simulink model "WESDem_CalcState"  (R2016b)
settings: configuration reference "CodeGenConfigSet" (kept outside this file)
values from neighbouring files (symbols this model uses):
  WESDem_stCfg_C = Calibration.Parameter    [init_WESDem_CalcState.m]
  WESDem_stCfgvalid_C = Calibration.Parameter    [init_WESDem_CalcState.m]
  WESDem_stCrCtlInhibActv_C = Calibration.Parameter    [init_WESDem_CalcState.m]
  WESDem_stMode_C = Calibration.Parameter    [init_WESDem_CalcState.m]
  WESDem_stModevalid_C = Calibration.Parameter    [init_WESDem_CalcState.m]
  WESDem_swtEnaStrtModChng_C = Calibration.Parameter    [init_WESDem_CalcState.m]
  WESDem_tiBlockAftStrt_C = Calibration.Parameter    [init_WESDem_CalcState.m]
  WESDem_tiNeutr_C = Calibration.Parameter    [init_WESDem_CalcState.m]
  WESDem_trqThresNTC_C = Calibration.Parameter    [init_WESDem_CalcState.m]
  WESDem_vInhibCrCUI_C = Calibration.Parameter    [init_WESDem_CalcState.m]
  WESDem_vMaxAcc0_C = Calibration.Parameter    [init_WESDem_CalcState.m]
  WESDem_vMaxAcc1_C = Calibration.Parameter    [init_WESDem_CalcState.m]
  WESDem_vMaxAcc2_C = Calibration.Parameter    [init_WESDem_CalcState.m]
  WESDem_vMaxAcc3_C = Calibration.Parameter    [init_WESDem_CalcState.m]
undefined symbols (not defined in the file or in its folder): CrCUI_BttnState_conv, CruiseCtl_State_conv, EISGov_num_conv, EngState_conv, WESDem_CalcState_DT
libraries: simulink x50, CXLib x32
(part 1 of 2)
settings Model: Creator=zhoukai  LastModifiedBy=zhoukai
settings ConfigSetRef: SourceLocation=Base Workspace

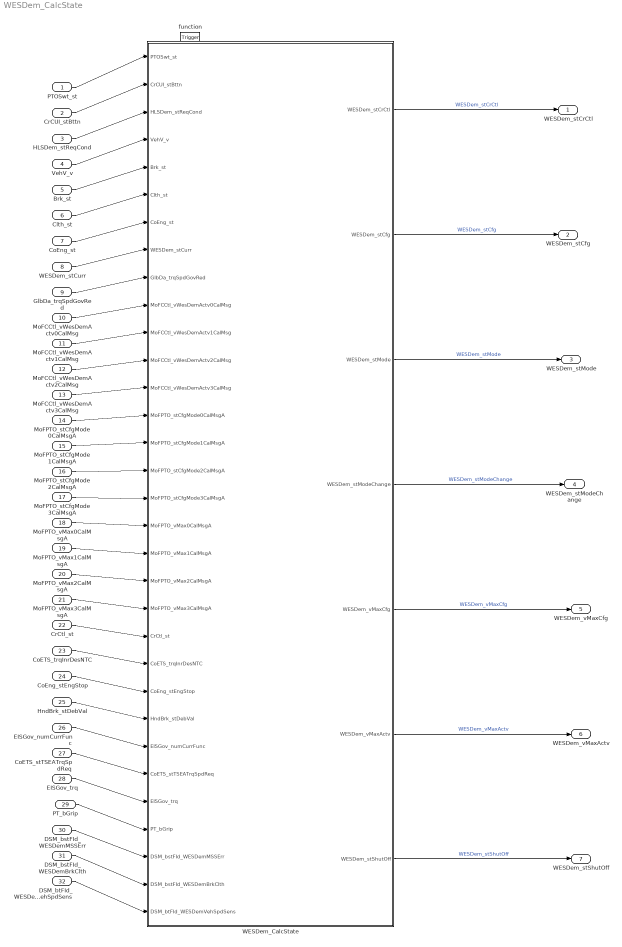
== system WESDem_CalcState ==
  PTOSwt_st : Inport  Description=Power Take-off switch's current state for a specific input voltage  OutMin=0  OutMax=255  OutDataTypeStr=State_uint8
  CrCUI_stBttn : Inport  Description=Application parameter for status button information  Port=2  OutDataTypeStr=Enum: CrCUI_BttnState_conv
  HLSDem_stReqCond : Inport  Description=Status of request for idle speed increase  Port=3  OutMin=0  OutMax=255  OutDataTypeStr=State_uint8
  VehV_v : Inport  Tag=km/h  Description=Vehicle speed  Port=4  OutMin=0  OutMax=250  OutDataTypeStr=VehSpeed_km_h
  Brk_st : Inport  Description=Brake switch state  Port=5  OutMin=0  OutMax=255  OutDataTypeStr=State_uint8
  Clth_st : Inport  Description=Clutch information  Port=6  OutMin=0  OutMax=255  OutDataTypeStr=State_uint8
  CoEng_st : Inport  Description=Engine coordinator state  Port=7  OutDataTypeStr=Enum: EngState_conv
  WESDem_stCurr : Inport  Description=Status of the working engine Speed Control  Port=8  OutDataTypeStr=Enum: WESDem_State_conv
  GlbDa_trqSpdGovRed : Inport  Tag=Nm  Description=Application parameter for negative torque threshold for the engine speed governor to be considered active.  Port=9  OutMin=-3276.8  OutMax=3276.7  OutDataTypeStr=Trq_Nm
  MoFCCtl_vWesDemActv0CalMsg : Inport  Tag=km/h  Description=MoFCCtl_vWesDemActvCalMsg[0]  Port=10  OutMin=0  OutMax=255  OutDataTypeStr=VehSpeed_km_h
  MoFCCtl_vWesDemActv1CalMsg : Inport  Tag=km/h  Description=MoFCCtl_vWesDemActvCalMsg[1]  Port=11  OutMin=0  OutMax=255  OutDataTypeStr=VehSpeed_km_h
  MoFCCtl_vWesDemActv2CalMsg : Inport  Tag=km/h  Description=MoFCCtl_vWesDemActvCalMsg[2]  Port=12  OutMin=0  OutMax=255  OutDataTypeStr=VehSpeed_km_h
  MoFCCtl_vWesDemActv3CalMsg : Inport  Tag=km/h  Description=MoFCCtl_vWesDemActvCalMsg[3]  Port=13  OutMin=0  OutMax=255  OutDataTypeStr=VehSpeed_km_h
  MoFPTO_stCfgMode0CalMsgA : Inport  Description=MoFPTO_stCfgModeCalMsgA[0]  Port=14  OutMin=0  OutMax=65535  OutDataTypeStr=State_uint16
  MoFPTO_stCfgMode1CalMsgA : Inport  Description=MoFPTO_stCfgModeCalMsgA[1]  Port=15  OutMin=0  OutMax=65535  OutDataTypeStr=State_uint16
  MoFPTO_stCfgMode2CalMsgA : Inport  Description=MoFPTO_stCfgModeCalMsgA[2]  Port=16  OutMin=0  OutMax=65535  OutDataTypeStr=State_uint16
  MoFPTO_stCfgMode3CalMsgA : Inport  Description=MoFPTO_stCfgModeCalMsgA[3]  Port=17  OutMin=0  OutMax=65535  OutDataTypeStr=State_uint16
  MoFPTO_vMax0CalMsgA : Inport  Tag=km/h  Description=MoFPTO_vMaxCalMsgA[0]  Port=18  OutMin=0  OutMax=250  OutDataTypeStr=VehSpeed_km_h
  MoFPTO_vMax1CalMsgA : Inport  Tag=km/h  Description=MoFPTO_vMaxCalMsgA[1]  Port=19  OutMin=0  OutMax=250  OutDataTypeStr=VehSpeed_km_h
  MoFPTO_vMax2CalMsgA : Inport  Tag=km/h  Description=MoFPTO_vMaxCalMsgA[2]  Port=20  OutMin=0  OutMax=250  OutDataTypeStr=VehSpeed_km_h
  MoFPTO_vMax3CalMsgA : Inport  Tag=km/h  Description=MoFPTO_vMaxCalMsgA[3]  Port=21  OutMin=0  OutMax=250  OutDataTypeStr=VehSpeed_km_h
  CrCtl_st : Inport  Description=Application parameter for Cruise Control state  Port=22  OutDataTypeStr=Enum: CruiseCtl_State_conv
  CoETS_trqInrDesNTC : Inport  Tag=Nm  Description=Additional desired engine friction Nm  Port=23  OutMin=-3276  OutMax=3276  OutDataTypeStr=Trq_Nm
  CoEng_stEngStop : Inport  Description=Bit coded output message from engine stop function for low idle, egine shut off and crank control  Port=24  OutMin=0  OutMax=255  OutDataTypeStr=State_uint8
  HndBrk_stDebVal : Inport  Description=Debounced value of Hand Brake switch  Port=25  OutMin=0  OutMax=255  OutDataTypeStr=State_uint8
  EISGov_numCurrFunc : Inport  Description=Identification name / number of the currently active EISGov client, which determines the current controller parameters  Port=26  OutDataTypeStr=Enum: EISGov_num_conv
  CoETS_stTSEATrqSpdReq : Inport  Description=Status of information about torque and speed intervention  Port=27  OutMin=0  OutMax=65535  OutDataTypeStr=State_uint16
  EISGov_trq : Inport  Tag=Nm  Description=Resulted output torque of EISGov controller  Port=28  OutMin=-3276.8  OutMax=3276.7  OutDataTypeStr=Trq_Nm
  PT_bGrip : Inport  Description=Grip is for sure present (the converter lockup clutch / the automated or manual clutch is completely closed and PT_bNoGrip = FALSE)  Port=29  OutMin=0  OutMax=1  OutDataTypeStr=boolean
  DSM_bstFId_WESDemMSSErr : Inport  Description=Function Identifier for WESDem reactions in case of multiple state switch error  Port=30  OutMin=0  OutMax=1  OutDataTypeStr=boolean
  DSM_bstFId_WESDemBrkClth : Inport  Description=FId inhibits if brake or clutch is faulty  Port=31  OutMin=0  OutMax=1  OutDataTypeStr=boolean
  DSM_btFId_WESDemVehSpdSens : Inport  Description=Function Identifier for WESDem reactions in case of vehicle speed sensing error  Port=32  OutMin=0  OutMax=1  OutDataTypeStr=boolean
  function : TriggerPort  TriggerType=function-call  VariantControl=Variant
  WESDem_CalcState : Subsystem
  WESDem_stCrCtl : Outport  Description=State control of the working engine speed demand  OutMin=0  OutMax=65535  OutDataTypeStr=State_uint16
  WESDem_stCfg : Outport  Description=Configuration of the actual operating mode  Port=2  OutMin=0  OutMax=65535  OutDataTypeStr=State_uint16
  WESDem_stMode : Outport  Description=Operating mode of the working engine speed demand  Port=3  OutMin=0  OutMax=255  OutDataTypeStr=State_uint8
  WESDem_stModeChange : Outport  Description=Operating mode change of the working engine speed demand  Port=4  OutMin=0  OutMax=255  OutDataTypeStr=State_uint8
  WESDem_vMaxCfg : Outport  Tag=km/h  Description=Maximum speed for activation in the actual operating mode  Port=5  OutMin=0  OutMax=255  OutDataTypeStr=VehSpeed_km_h
  WESDem_vMaxActv : Outport  Tag=km/h  Description=Vehicle speed threshold for activation of the WESDem  Port=6  OutMin=0  OutMax=255  OutDataTypeStr=VehSpeed_km_h
  WESDem_stShutOff : Outport  Description=Shut off conditions for the Working engine speed Demand  Port=7  OutMin=0  OutMax=65535  OutDataTypeStr=State_uint16
  wires:
  PTOSwt_st/1 -> WESDem_CalcState/1(PTOSwt_st)
  CrCUI_stBttn/1 -> WESDem_CalcState/2(CrCUI_stBttn)
  HLSDem_stReqCond/1 -> WESDem_CalcState/3(HLSDem_stReqCond)
  VehV_v/1 -> WESDem_CalcState/4(VehV_v)
  Brk_st/1 -> WESDem_CalcState/5(Brk_st)
  Clth_st/1 -> WESDem_CalcState/6(Clth_st)
  CoEng_st/1 -> WESDem_CalcState/7(CoEng_st)
  WESDem_stCurr/1 -> WESDem_CalcState/8(WESDem_stCurr)
  GlbDa_trqSpdGovRed/1 -> WESDem_CalcState/9(GlbDa_trqSpdGovRed)
  MoFCCtl_vWesDemActv0CalMsg/1 -> WESDem_CalcState/10(MoFCCtl_vWesDemActv0CalMsg)
  MoFCCtl_vWesDemActv1CalMsg/1 -> WESDem_CalcState/11(MoFCCtl_vWesDemActv1CalMsg)
  MoFCCtl_vWesDemActv2CalMsg/1 -> WESDem_CalcState/12(MoFCCtl_vWesDemActv2CalMsg)
  MoFCCtl_vWesDemActv3CalMsg/1 -> WESDem_CalcState/13(MoFCCtl_vWesDemActv3CalMsg)
  MoFPTO_stCfgMode0CalMsgA/1 -> WESDem_CalcState/14(MoFPTO_stCfgMode0CalMsgA)
  MoFPTO_stCfgMode1CalMsgA/1 -> WESDem_CalcState/15(MoFPTO_stCfgMode1CalMsgA)
  MoFPTO_stCfgMode2CalMsgA/1 -> WESDem_CalcState/16(MoFPTO_stCfgMode2CalMsgA)
  MoFPTO_stCfgMode3CalMsgA/1 -> WESDem_CalcState/17(MoFPTO_stCfgMode3CalMsgA)
  MoFPTO_vMax0CalMsgA/1 -> WESDem_CalcState/18(MoFPTO_vMax0CalMsgA)
  MoFPTO_vMax1CalMsgA/1 -> WESDem_CalcState/19(MoFPTO_vMax1CalMsgA)
  MoFPTO_vMax2CalMsgA/1 -> WESDem_CalcState/20(MoFPTO_vMax2CalMsgA)
  MoFPTO_vMax3CalMsgA/1 -> WESDem_CalcState/21(MoFPTO_vMax3CalMsgA)
  CrCtl_st/1 -> WESDem_CalcState/22(CrCtl_st)
  CoETS_trqInrDesNTC/1 -> WESDem_CalcState/23(CoETS_trqInrDesNTC)
  CoEng_stEngStop/1 -> WESDem_CalcState/24(CoEng_stEngStop)
  HndBrk_stDebVal/1 -> WESDem_CalcState/25(HndBrk_stDebVal)
  EISGov_numCurrFunc/1 -> WESDem_CalcState/26(EISGov_numCurrFunc)
  CoETS_stTSEATrqSpdReq/1 -> WESDem_CalcState/27(CoETS_stTSEATrqSpdReq)
  EISGov_trq/1 -> WESDem_CalcState/28(EISGov_trq)
  PT_bGrip/1 -> WESDem_CalcState/29(PT_bGrip)
  WESDem_CalcState/1(WESDem_stCrCtl) -> WESDem_stCrCtl/1  "WESDem_stCrCtl"
  WESDem_CalcState/2(WESDem_stCfg) -> WESDem_stCfg/1  "WESDem_stCfg"
  WESDem_CalcState/3(WESDem_stMode) -> WESDem_stMode/1  "WESDem_stMode"
  WESDem_CalcState/4(WESDem_stModeChange) -> WESDem_stModeChange/1  "WESDem_stModeChange"
  WESDem_CalcState/5(WESDem_vMaxCfg) -> WESDem_vMaxCfg/1  "WESDem_vMaxCfg"
  WESDem_CalcState/6(WESDem_vMaxActv) -> WESDem_vMaxActv/1  "WESDem_vMaxActv"
  WESDem_CalcState/7(WESDem_stShutOff) -> WESDem_stShutOff/1  "WESDem_stShutOff"
  DSM_bstFId_WESDemMSSErr/1 -> WESDem_CalcState/30("DSM_bstFId_WESDemMSSErr ")
  DSM_bstFId_WESDemBrkClth/1 -> WESDem_CalcState/31("DSM_bstFId_WESDemBrkClth ")
  DSM_btFId_WESDemVehSpdSens/1 -> WESDem_CalcState/32("DSM_btFId_WESDemVehSpdSens ")

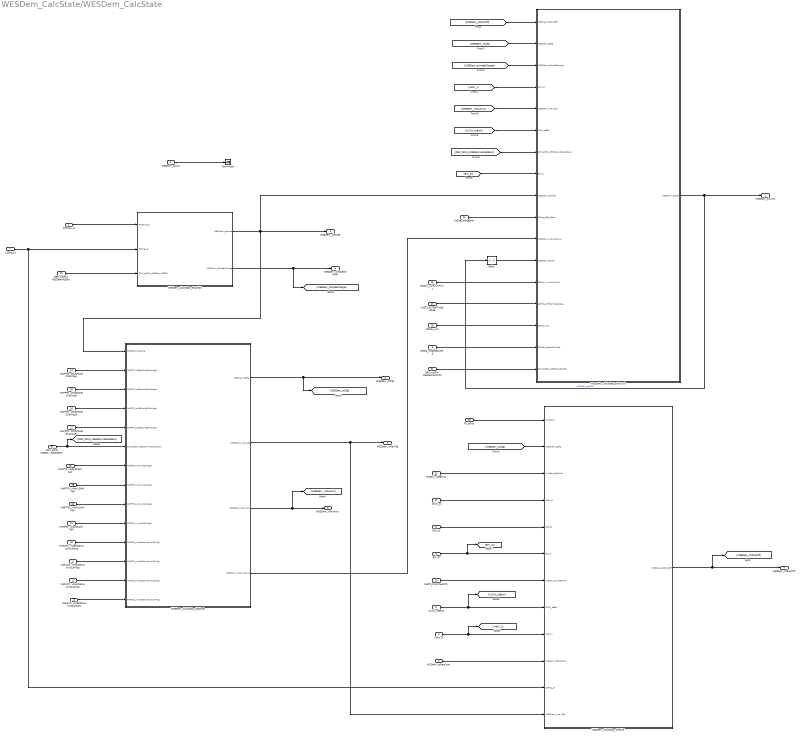
== system WESDem_CalcState/WESDem_CalcState ==
  PTOSwt_st : Inport  Description=Power Take-off switch's current state for a specific input voltage  OutMin=0  OutMax=255  OutDataTypeStr=State_uint8
  CrCUI_stBttn : Inport  Description=Application parameter for status button information  Port=2
  HLSDem_stReqCond : Inport  Description=Status of request for idle speed increase  Port=3  OutMin=0  OutMax=255  OutDataTypeStr=State_uint8
  VehV_v : Inport  Tag=km/h  Description=Vehicle speed  Port=4  OutMin=0  OutMax=250  OutDataTypeStr=VehSpeed_km_h
  Brk_st : Inport  Description=Brake switch state  Port=5  OutMin=0  OutMax=255  OutDataTypeStr=State_uint8
  Clth_st : Inport  Description=Clutch information  Port=6  OutMin=0  OutMax=255  OutDataTypeStr=State_uint8
  CoEng_st : Inport  Description=Engine coordinator state  Port=7  OutDataTypeStr=Enum: EngState_conv
  WESDem_stCurr : Inport  Description=Status of the working engine Speed Control  Port=8  OutDataTypeStr=Enum: WESDem_State_conv
  GlbDa_trqSpdGovRed : Inport  Tag=Nm  Description=Application parameter for negative torque threshold for the engine speed governor to be considered active.  Port=9  OutMin=-3276.8  OutMax=3276.7  OutDataTypeStr=Trq_Nm
  MoFCCtl_vWesDemActv0CalMsg : Inport  Tag=km/h  Description=MoFCCtl_vWesDemActvCalMsg[0]  Port=10  OutMin=0  OutMax=255  OutDataTypeStr=VehSpeed_km_h
  MoFCCtl_vWesDemActv1CalMsg : Inport  Tag=km/h  Description=MoFCCtl_vWesDemActvCalMsg[1]  Port=11  OutMin=0  OutMax=255  OutDataTypeStr=VehSpeed_km_h
  MoFCCtl_vWesDemActv2CalMsg : Inport  Tag=km/h  Description=MoFCCtl_vWesDemActvCalMsg[2]  Port=12  OutMin=0  OutMax=255  OutDataTypeStr=VehSpeed_km_h
  MoFCCtl_vWesDemActv3CalMsg : Inport  Tag=km/h  Description=MoFCCtl_vWesDemActvCalMsg[3]  Port=13  OutMin=0  OutMax=255  OutDataTypeStr=VehSpeed_km_h
  MoFPTO_stCfgMode0CalMsgA : Inport  Description=MoFPTO_stCfgModeCalMsgA[0]  Port=14  OutMin=0  OutMax=65535  OutDataTypeStr=State_uint16
  MoFPTO_stCfgMode1CalMsgA : Inport  Description=MoFPTO_stCfgModeCalMsgA[1]  Port=15  OutMin=0  OutMax=65535  OutDataTypeStr=State_uint16
  MoFPTO_stCfgMode2CalMsgA : Inport  Description=MoFPTO_stCfgModeCalMsgA[2]  Port=16  OutMin=0  OutMax=65535  OutDataTypeStr=State_uint16
  MoFPTO_stCfgMode3CalMsgA : Inport  Description=MoFPTO_stCfgModeCalMsgA[3]  Port=17  OutMin=0  OutMax=65535  OutDataTypeStr=State_uint16
  MoFPTO_vMax0CalMsgA : Inport  Tag=km/h  Description=MoFPTO_vMaxCalMsgA[0]  Port=18  OutMin=0  OutMax=250  OutDataTypeStr=VehSpeed_km_h
  MoFPTO_vMax1CalMsgA : Inport  Tag=km/h  Description=MoFPTO_vMaxCalMsgA[1]  Port=19  OutMin=0  OutMax=250  OutDataTypeStr=VehSpeed_km_h
  MoFPTO_vMax2CalMsgA : Inport  Tag=km/h  Description=MoFPTO_vMaxCalMsgA[2]  Port=20  OutMin=0  OutMax=250  OutDataTypeStr=VehSpeed_km_h
  MoFPTO_vMax3CalMsgA : Inport  Tag=km/h  Description=MoFPTO_vMaxCalMsgA[3]  Port=21  OutMin=0  OutMax=250  OutDataTypeStr=VehSpeed_km_h
  CrCtl_st : Inport  Description=Application parameter for Cruise Control state  Port=22
  CoETS_trqInrDesNTC : Inport  Tag=Nm  Description=Additional desired engine friction Nm  Port=23  OutMin=-3276  OutMax=3276  OutDataTypeStr=Trq_Nm
  CoEng_stEngStop : Inport  Description=Bit coded output message from engine stop function for low idle, egine shut off and crank control  Port=24  OutMin=0  OutMax=255  OutDataTypeStr=State_uint8
  HndBrk_stDebVal : Inport  Description=Debounced value of Hand Brake switch  Port=25  OutMin=0  OutMax=255  OutDataTypeStr=State_uint8
  EISGov_numCurrFunc : Inport  Description=Identification name / number of the currently active EISGov client, which determines the current controller parameters  Port=26  OutDataTypeStr=Enum: EISGov_num_conv
  CoETS_stTSEATrqSpdReq : Inport  Description=Status of information about torque and speed intervention  Port=27  OutMin=0  OutMax=65535  OutDataTypeStr=State_uint16
  EISGov_trq : Inport  Tag=Nm  Description=Resulted output torque of EISGov controller  Port=28  OutMin=-3276.8  OutMax=3276.7  OutDataTypeStr=Trq_Nm
  PT_bGrip : Inport  Description=Grip is for sure present (the converter lockup clutch / the automated or manual clutch is completely closed and PT_bNoGrip = FALSE)  Port=29  OutMin=0  OutMax=1  OutDataTypeStr=boolean
  "DSM_bstFId_WESDemMSSErr " : Inport  Description=Function Identifier for WESDem reactions in case of multiple state switch error  Port=30  OutMin=0  OutMax=1  OutDataTypeStr=boolean
  "DSM_bstFId_WESDemBrkClth " : Inport  Description=FId inhibits if brake or clutch is faulty  Port=31  OutMin=0  OutMax=1  OutDataTypeStr=boolean
  "DSM_btFId_WESDemVehSpdSens " : Inport  Description=Function Identifier for WESDem reactions in case of vehicle speed sensing error  Port=32  OutMin=0  OutMax=1  OutDataTypeStr=boolean
  Delay : Delay  DelayLength=1  InitialCondition=0
  Terminator : Terminator
  WESDem_CalcState_CfgMode : Subsystem
  WESDem_CalcState_EvalCrCtl : Subsystem
  WESDem_CalcState_EvalMSS : Subsystem
  WESDem_CalcState_ShutOff : Subsystem
  WESDem_stCrCtl : Outport  Description=State control of the working engine speed demand  OutMin=0  OutMax=65535  OutDataTypeStr=State_uint16
  WESDem_stCfg : Outport  Description=Configuration of the actual operating mode  Port=2  OutMin=0  OutMax=65535  OutDataTypeStr=State_uint16
  WESDem_stMode : Outport  Description=Operating mode of the working engine speed demand  Port=3  OutMin=0  OutMax=255  OutDataTypeStr=State_uint8
  WESDem_stModeChange : Outport  Description=Operating mode change of the working engine speed demand  Port=4  OutMin=0  OutMax=255  OutDataTypeStr=State_uint8
  WESDem_vMaxCfg : Outport  Description=Maximum speed for activation in the actual operating mode  Port=5  OutMin=0  OutMax=255  OutDataTypeStr=VehSpeed_km_h
  WESDem_vMaxActv : Outport  Description=Vehicle speed threshold for activation of the WESDem  Port=6  OutMin=0  OutMax=255  OutDataTypeStr=VehSpeed_km_h
  WESDem_stShutOff : Outport  Description=Shut off conditions for the Working engine speed Demand  Port=7  OutMin=0  OutMax=65535  OutDataTypeStr=State_uint16
  wires:
  WESDem_CalcState_EvalCrCtl/1(WESDem_stCrCtl) -> Delay/1, WESDem_stCrCtl/1  "WESDem_stCrCtl"
  PTOSwt_st/1 -> WESDem_CalcState_EvalMSS/1(PTOSwt_st)
  WESDem_CalcState_EvalMSS/2(WESDem_stModeChange) -> [WESDem_stModeChange], WESDem_stModeChange/1
  MoFPTO_stCfgMode0CalMsgA/1 -> WESDem_CalcState_CfgMode/2(MoFPTO_stCfgMode0CalMsgA)
  MoFPTO_stCfgMode1CalMsgA/1 -> WESDem_CalcState_CfgMode/3(MoFPTO_stCfgMode1CalMsgA)
  MoFPTO_stCfgMode2CalMsgA/1 -> WESDem_CalcState_CfgMode/4(MoFPTO_stCfgMode2CalMsgA)
  MoFPTO_stCfgMode3CalMsgA/1 -> WESDem_CalcState_CfgMode/5(MoFPTO_stCfgMode3CalMsgA)
  "DSM_btFId_WESDemVehSpdSens "/1 -> [DSM_btFId_WESDemVehSpdSens], WESDem_CalcState_CfgMode/6("DSM_btFId_WESDemVehSpdSens ")
  MoFPTO_vMax0CalMsgA/1 -> WESDem_CalcState_CfgMode/7(MoFPTO_vMax0CalMsgA)
  MoFPTO_vMax1CalMsgA/1 -> WESDem_CalcState_CfgMode/8(MoFPTO_vMax1CalMsgA)
  MoFPTO_vMax2CalMsgA/1 -> WESDem_CalcState_CfgMode/9(MoFPTO_vMax2CalMsgA)
  MoFPTO_vMax3CalMsgA/1 -> WESDem_CalcState_CfgMode/10(MoFPTO_vMax3CalMsgA)
  MoFCCtl_vWesDemActv0CalMsg/1 -> WESDem_CalcState_CfgMode/11(MoFCCtl_vWesDemActv0CalMsg)
  MoFCCtl_vWesDemActv1CalMsg/1 -> WESDem_CalcState_CfgMode/12(MoFCCtl_vWesDemActv1CalMsg)
  MoFCCtl_vWesDemActv2CalMsg/1 -> WESDem_CalcState_CfgMode/13(MoFCCtl_vWesDemActv2CalMsg)
  MoFCCtl_vWesDemActv3CalMsg/1 -> WESDem_CalcState_CfgMode/14(MoFCCtl_vWesDemActv3CalMsg)
  WESDem_CalcState_CfgMode/1(WESDem_stCfg) -> [WESDem_stCfg], WESDem_stCfg/1
  WESDem_CalcState_CfgMode/2(WESDem_vMaxCfg) -> WESDem_CalcState_ShutOff/12(WESDem_vMaxCfg), WESDem_vMaxCfg/1
  WESDem_CalcState_CfgMode/3(WESDem_vMaxActv) -> [WESDem_vMaxActv], WESDem_vMaxActv/1
  WESDem_CalcState_EvalMSS/1(WESDem_stMode) -> WESDem_CalcState_EvalCrCtl/9("WESDem_stMode "), WESDem_CalcState_CfgMode/1(WESDem_stMode), WESDem_stMode/1
  CoEng_st/1 -> WESDem_CalcState_ShutOff/11(CoEng_st), WESDem_CalcState_EvalMSS/2(CoEng_st)
  HndBrk_stDebVal/1 -> WESDem_CalcState_ShutOff/3(HndBrk_stDebVal)
  CrCtl_st/1 -> WESDem_CalcState_ShutOff/4(CrCtl_st)
  Clth_st/1 -> WESDem_CalcState_ShutOff/5(Clth_st)
  Brk_st/1 -> [Brk_st], WESDem_CalcState_ShutOff/6(Brk_st)
  CoETS_trqInrDesNTC/1 -> WESDem_CalcState_ShutOff/7(CoETS_trqInrDesNTC)
  CrCUI_stBttn/1 -> [CrCUI_stBttn], WESDem_CalcState_ShutOff/8(CrCUI_stBttn)
  VehV_v/1 -> [VehV_v], WESDem_CalcState_ShutOff/9(VehV_v)
  HLSDem_stReqCond/1 -> WESDem_CalcState_ShutOff/10(HLSDem_stReqCond)
  WESDem_CalcState_ShutOff/1(WESDem_stShutOff) -> [WESDem_stShutOff], WESDem_stShutOff/1
  PT_bGrip/1 -> WESDem_CalcState_ShutOff/1(PT_bGrip)
  GlbDa_trqSpdGovRed/1 -> WESDem_CalcState_EvalCrCtl/16(GlbDa_trqSpdGovRed)
  EISGov_trq/1 -> WESDem_CalcState_EvalCrCtl/15(EISGov_trq)
  CoETS_stTSEATrqSpdReq/1 -> WESDem_CalcState_EvalCrCtl/14(CoETS_stTSEATrqSpdReq)
  EISGov_numCurrFunc/1 -> WESDem_CalcState_EvalCrCtl/13("EISGov_numCurrFunc ")
  CoEng_stEngStop/1 -> WESDem_CalcState_EvalCrCtl/10(CoEng_stEngStop)
  WESDem_stCurr/1 -> Terminator/1
  [WESDem_stShutOff] -> WESDem_CalcState_EvalCrCtl/1(WESDem_stShutOff)
  [WESDem_stCfg] -> WESDem_CalcState_EvalCrCtl/2(WESDem_stCfg)
  [WESDem_stCfg] -> WESDem_CalcState_ShutOff/2(WESDem_stCfg)
  [WESDem_stModeChange] -> WESDem_CalcState_EvalCrCtl/3(WESDem_stModeChange)
  [VehV_v] -> WESDem_CalcState_EvalCrCtl/4(VehV_v)
  [WESDem_vMaxActv] -> WESDem_CalcState_EvalCrCtl/5(WESDem_vMaxActv)
  [CrCUI_stBttn] -> WESDem_CalcState_EvalCrCtl/6(CrCUI_stBttn)
  [DSM_btFId_WESDemVehSpdSens] -> WESDem_CalcState_EvalCrCtl/7("DSM_btFId_WESDemVehSpdSens ")
  [Brk_st] -> WESDem_CalcState_EvalCrCtl/8(Brk_st)
  Delay/1 -> WESDem_CalcState_EvalCrCtl/12("WESDem_stCrCtl ")
  WESDem_CalcState_CfgMode/4(WESDem_vMaxAcc_mp) -> WESDem_CalcState_EvalCrCtl/11("WESDem_vMaxAcc_mp ")
  "DSM_bstFId_WESDemMSSErr "/1 -> WESDem_CalcState_EvalMSS/3("DSM_bstFId_WESDemMSSErr ")
  "DSM_bstFId_WESDemBrkClth "/1 -> WESDem_CalcState_EvalCrCtl/17("DSM_bstFId_WESDemBrkClth ")

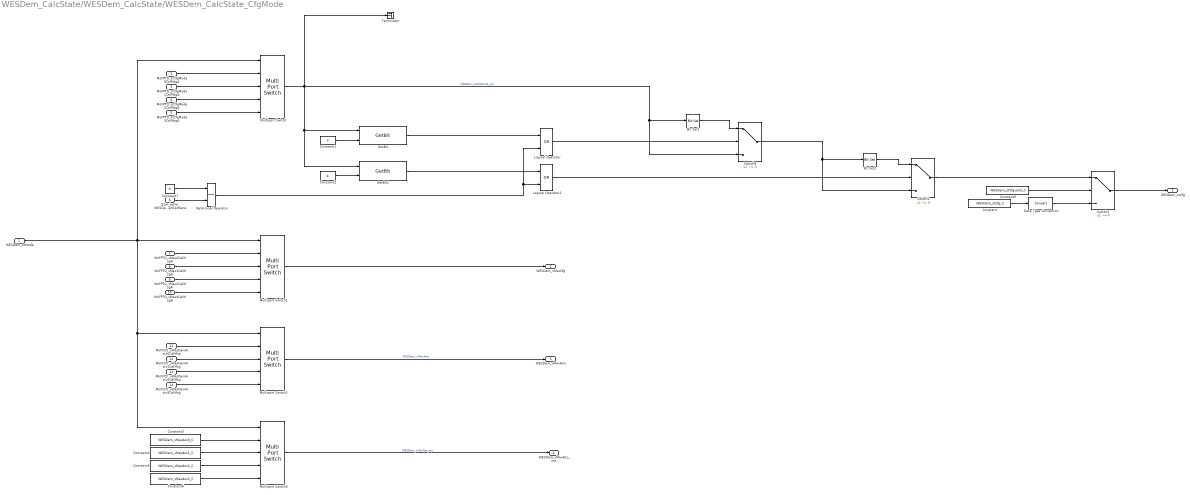
== system WESDem_CalcState/WESDem_CalcState/WESDem_CalcState_CfgMode ==
  WESDem_stMode : Inport  Tag=km/h  Description=MoFPTO_vMaxCalMsgA[0]  OutMin=0  OutMax=250  OutDataTypeStr=uint8
  MoFPTO_stCfgMode0CalMsgA : Inport  Description=MoFPTO_stCfgModeCalMsgA[0]  Port=2  OutMin=0  OutMax=65535  OutDataTypeStr=State_uint16
  MoFPTO_stCfgMode1CalMsgA : Inport  Description=MoFPTO_stCfgModeCalMsgA[1]  Port=3  OutMin=0  OutMax=65535  OutDataTypeStr=State_uint16
  MoFPTO_stCfgMode2CalMsgA : Inport  Description=MoFPTO_stCfgModeCalMsgA[2]  Port=4  OutMin=0  OutMax=65535  OutDataTypeStr=State_uint16
  MoFPTO_stCfgMode3CalMsgA : Inport  Description=MoFPTO_stCfgModeCalMsgA[3]  Port=5  OutMin=0  OutMax=65535  OutDataTypeStr=State_uint16
  "DSM_btFId_WESDemVehSpdSens " : Inport  Description=Function Identifier for WESDem reactions in case of vehicle speed sensing error  Port=6  OutMin=0  OutMax=1  OutDataTypeStr=boolean
  MoFPTO_vMax0CalMsgA : Inport  Tag=km/h  Description=MoFPTO_vMaxCalMsgA[0]  Port=7  OutMin=0  OutMax=250  OutDataTypeStr=VehSpeed_km_h
  MoFPTO_vMax1CalMsgA : Inport  Tag=km/h  Description=MoFPTO_vMaxCalMsgA[1]  Port=8  OutMin=0  OutMax=250  OutDataTypeStr=VehSpeed_km_h
  MoFPTO_vMax2CalMsgA : Inport  Tag=km/h  Description=MoFPTO_vMaxCalMsgA[2]  Port=9  OutMin=0  OutMax=250  OutDataTypeStr=VehSpeed_km_h
  MoFPTO_vMax3CalMsgA : Inport  Tag=km/h  Description=MoFPTO_vMaxCalMsgA[3]  Port=10  OutMin=0  OutMax=250  OutDataTypeStr=VehSpeed_km_h
  MoFCCtl_vWesDemActv0CalMsg : Inport  Tag=km/h  Description=MoFCCtl_vWesDemActvCalMsg[0]  Port=11  OutMin=0  OutMax=255  OutDataTypeStr=VehSpeed_km_h
  MoFCCtl_vWesDemActv1CalMsg : Inport  Tag=km/h  Description=MoFCCtl_vWesDemActvCalMsg[1]  Port=12  OutMin=0  OutMax=255  OutDataTypeStr=VehSpeed_km_h
  MoFCCtl_vWesDemActv2CalMsg : Inport  Tag=km/h  Description=MoFCCtl_vWesDemActvCalMsg[2]  Port=13  OutMin=0  OutMax=255  OutDataTypeStr=VehSpeed_km_h
  MoFCCtl_vWesDemActv3CalMsg : Inport  Tag=km/h  Description=MoFCCtl_vWesDemActvCalMsg[3]  Port=14  OutMin=0  OutMax=255  OutDataTypeStr=VehSpeed_km_h
  Bit Set1 : simulink/Logic and Bit Operations/Bit Set  iBit=3
  Bit Set2 : simulink/Logic and Bit Operations/Bit Set  iBit=4
  Constant : Constant  Value=WESDem_stCfg_C
  Constant1 : Constant  Value=3  OutDataTypeStr=Inherit: Inherit via back propagation
  Constant2 : Constant  Value=4  OutDataTypeStr=Inherit: Inherit via back propagation
  Constant3 : Constant  Value=WESDem_vMaxAcc0_C
  Constant4 : Constant  Value=WESDem_vMaxAcc1_C
  Constant5 : Constant  Value=WESDem_vMaxAcc2_C
  Constant6 : Constant  Value=WESDem_vMaxAcc3_C
  Constant7 : Constant  Value=0  OutDataTypeStr=Inherit: Inherit via back propagation
  Constant9 : Constant  Value=WESDem_stCfgvalid_C
  Data Type Conversion : DataTypeConversion
  GetBit : CXLib/GetBit  dataTypeString=uint16  dataLength=0
      settings: AttributesFormatString=Get bit from %<dataTypeString>
  GetBit1 : CXLib/GetBit  dataTypeString=uint16  dataLength=0
      settings: AttributesFormatString=Get bit from %<dataTypeString>
  Logical Operator : Logic  Operator=OR  AllPortsSameDT=off  OutDataTypeStr=boolean
  Logical Operator1 : Logic  Operator=OR  AllPortsSameDT=off  OutDataTypeStr=boolean
  Multiport Switch{,1..3} (4 alike) : MultiPortSwitch  DataPortOrder=Zero-based contiguous  Inputs=4
  Relational Operator : RelationalOperator  Operator===  OutDataTypeStr=boolean  RndMeth=Simplest
  Switch1 : Switch  Criteria=u2 ~= 0
  Switch2 : Switch  Criteria=u2 ~= 0
  Switch8 : Switch  Criteria=u2 ~= 0
  Terminator : Terminator
  WESDem_stCfg : Outport  Description=Configuration of the actual operating mode  OutMin=0  OutMax=65535  OutDataTypeStr=State_uint16
  WESDem_vMaxCfg : Outport  Description=Maximum speed for activation in the actual operating mode  Port=2  OutMin=0  OutMax=255  OutDataTypeStr=VehSpeed_km_h
  WESDem_vMaxActv : Outport  Description=Vehicle speed threshold for activation of the WESDem  Port=3  OutMin=0  OutMax=255  OutDataTypeStr=VehSpeed_km_h
  WESDem_vMaxAcc_mp : Outport  Description=Vehicle speed threshold for activation of the WESDem  Port=4  OutMin=0  OutMax=250  OutDataTypeStr=VehSpeed_km_h
  wires:
  Multiport Switch1/1 -> WESDem_vMaxCfg/1
  Multiport Switch2/1 -> WESDem_vMaxActv/1  "WESDem_vMaxActv"
  MoFCCtl_vWesDemActv2CalMsg/1 -> Multiport Switch2/4
  Constant6/1 -> Multiport Switch3/5
  Constant1/1 -> GetBit/2
  MoFPTO_stCfgMode2CalMsgA/1 -> Multiport Switch/4
  MoFPTO_stCfgMode1CalMsgA/1 -> Multiport Switch/3
  MoFPTO_vMax3CalMsgA/1 -> Multiport Switch1/5
  MoFPTO_vMax1CalMsgA/1 -> Multiport Switch1/3
  MoFPTO_stCfgMode0CalMsgA/1 -> Multiport Switch/2
  MoFPTO_stCfgMode3CalMsgA/1 -> Multiport Switch/5
  Multiport Switch/1 -> Switch8/3, Bit Set1/1, Terminator/1, GetBit1/1, GetBit/1  "WESDem_stCfgMode_mp"
  Constant2/1 -> GetBit1/2
  Multiport Switch3/1 -> WESDem_vMaxAcc_mp/1  "WESDem_vMaxAcc_mp"
  MoFPTO_vMax0CalMsgA/1 -> Multiport Switch1/2
  Constant3/1 -> Multiport Switch3/2
  Constant4/1 -> Multiport Switch3/3
  MoFCCtl_vWesDemActv3CalMsg/1 -> Multiport Switch2/5
  Constant5/1 -> Multiport Switch3/4
  MoFCCtl_vWesDemActv0CalMsg/1 -> Multiport Switch2/2
  MoFCCtl_vWesDemActv1CalMsg/1 -> Multiport Switch2/3
  MoFPTO_vMax2CalMsgA/1 -> Multiport Switch1/4
  WESDem_stMode/1 -> Multiport Switch3/1, Multiport Switch2/1, Multiport Switch1/1, Multiport Switch/1
  GetBit1/1 -> Logical Operator1/1
  GetBit/1 -> Logical Operator/1
  Logical Operator/1 -> Switch8/2
  Logical Operator1/1 -> Switch1/2
  Relational Operator/1 -> Logical Operator/2, Logical Operator1/2
  Switch8/1 -> Switch1/3, Bit Set2/1
  Switch1/1 -> Switch2/1
  Switch2/1 -> WESDem_stCfg/1
  Constant/1 -> Data Type Conversion/1
  Data Type Conversion/1 -> Switch2/3
  Constant9/1 -> Switch2/2
  "DSM_btFId_WESDemVehSpdSens "/1 -> Relational Operator/2
  Constant7/1 -> Relational Operator/1
  Bit Set1/1 -> Switch8/1
  Bit Set2/1 -> Switch1/1

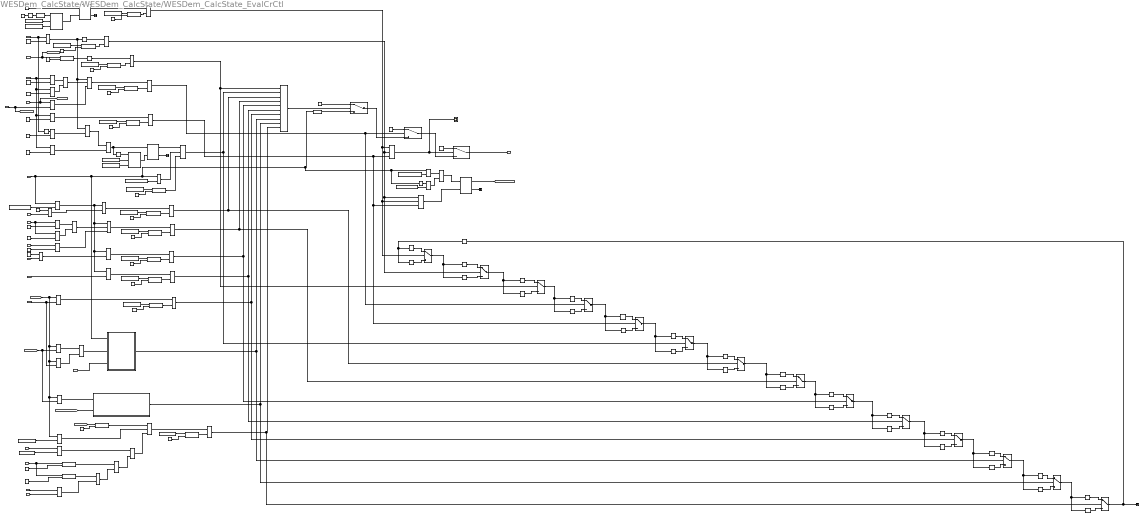
== system WESDem_CalcState/WESDem_CalcState/WESDem_CalcState_EvalCrCtl ==
  WESDem_stShutOff : Inport  Description=Application parameter for status button information  OutMin=0  OutMax=65535  OutDataTypeStr=uint16
  WESDem_stCfg : Inport  Description=Application parameter for status button information  Port=2  OutMin=0  OutMax=65535  OutDataTypeStr=uint16
  WESDem_stModeChange : Inport  Description=Application parameter for status button information  Port=3  OutMin=0  OutMax=255  OutDataTypeStr=uint8
  VehV_v : Inport  Tag=km/h  Description=Vehicle speed  Port=4  OutMin=0  OutMax=250  OutDataTypeStr=VehSpeed_km_h
  WESDem_vMaxActv : Inport  Description=Application parameter for status button information  Port=5  OutMin=0  OutMax=255  OutDataTypeStr=VehSpeed_km_h
  CrCUI_stBttn : Inport  Description=Application parameter for status button information  Port=6
  "DSM_btFId_WESDemVehSpdSens " : Inport  Description=Function Identifier for WESDem reactions in case of vehicle speed sensing error  Port=7  OutMin=0  OutMax=1  OutDataTypeStr=boolean
  Brk_st : Inport  Description=Brake switch state  Port=8  OutMin=0  OutMax=255  OutDataTypeStr=State_uint8
  "WESDem_stMode " : Inport  Description=Brake switch state  Port=9  OutMin=0  OutMax=255  OutDataTypeStr=State_uint8
  CoEng_stEngStop : Inport  Description=Bit coded output message from engine stop function for low idle, egine shut off and crank control  Port=10  OutMin=0  OutMax=255  OutDataTypeStr=State_uint8
  "WESDem_vMaxAcc_mp " : Inport  Description=Bit coded output message from engine stop function for low idle, egine shut off and crank control  Port=11  OutMin=0  OutMax=250  OutDataTypeStr=VehSpeed_km_h
  "WESDem_stCrCtl " : Inport  Description=Bit coded output message from engine stop function for low idle, egine shut off and crank control  Port=12  OutMin=0  OutMax=65535  OutDataTypeStr=uint16
  "EISGov_numCurrFunc " : Inport  Description=Engine coordinator state  Port=13  OutDataTypeStr=Enum: EISGov_num_conv
  CoETS_stTSEATrqSpdReq : Inport  Description=Status of information about torque and speed intervention  Port=14  OutMin=0  OutMax=65535  OutDataTypeStr=State_uint16
  EISGov_trq : Inport  Tag=Nm  Description=Resulted output torque of EISGov controller  Port=15  OutMin=-3276.8  OutMax=3276.7  OutDataTypeStr=Trq_Nm
  GlbDa_trqSpdGovRed : Inport  Tag=Nm  Description=Application parameter for negative torque threshold for the engine speed governor to be considered active.  Port=16  OutMin=-3276.8  OutMax=3276.7  OutDataTypeStr=Trq_Nm
  "DSM_bstFId_WESDemBrkClth " : Inport  Description=FId inhibits if brake or clutch is faulty  Port=17  OutMin=0  OutMax=1  OutDataTypeStr=boolean
  Bit Clear : simulink/Logic and Bit Operations/Bit Clear  iBit=0
  Bit Clear1 : simulink/Logic and Bit Operations/Bit Clear  iBit=1
  Bit Clear10 : simulink/Logic and Bit Operations/Bit Clear  iBit=10
  Bit Clear11 : simulink/Logic and Bit Operations/Bit Clear  iBit=11
  Bit Clear12 : simulink/Logic and Bit Operations/Bit Clear  iBit=12
  Bit Clear13 : simulink/Logic and Bit Operations/Bit Clear  iBit=13
  Bit Clear2 : simulink/Logic and Bit Operations/Bit Clear  iBit=2
  Bit Clear3 : simulink/Logic and Bit Operations/Bit Clear  iBit=3
  Bit Clear4 : simulink/Logic and Bit Operations/Bit Clear  iBit=4
  Bit Clear5 : simulink/Logic and Bit Operations/Bit Clear  iBit=5
  Bit Clear6 : simulink/Logic and Bit Operations/Bit Clear  iBit=6
  Bit Clear7 : simulink/Logic and Bit Operations/Bit Clear  iBit=7
  Bit Clear8 : simulink/Logic and Bit Operations/Bit Clear  iBit=8
  Bit Clear9 : simulink/Logic and Bit Operations/Bit Clear  iBit=9
  Bit Set : simulink/Logic and Bit Operations/Bit Set  iBit=0
  Bit Set1 : simulink/Logic and Bit Operations/Bit Set  iBit=1
  Bit Set10 : simulink/Logic and Bit Operations/Bit Set  iBit=10
  Bit Set11 : simulink/Logic and Bit Operations/Bit Set  iBit=11
  Bit Set12 : simulink/Logic and Bit Operations/Bit Set  iBit=12
  Bit Set13 : simulink/Logic and Bit Operations/Bit Set  iBit=13
  Bit Set2 : simulink/Logic and Bit Operations/Bit Set  iBit=2
  Bit Set3 : simulink/Logic and Bit Operations/Bit Set  iBit=3
  Bit Set4 : simulink/Logic and Bit Operations/Bit Set  iBit=4
  Bit Set5 : simulink/Logic and Bit Operations/Bit Set  iBit=5
  Bit Set6 : simulink/Logic and Bit Operations/Bit Set  iBit=6
  Bit Set7 : simulink/Logic and Bit Operations/Bit Set  iBit=7
  Bit Set8 : simulink/Logic and Bit Operations/Bit Set  iBit=8
  Bit Set9 : simulink/Logic and Bit Operations/Bit Set  iBit=9
  Constant{,1,7..8,11,28,51} (7 alike) : Constant  OutDataTypeStr=Inherit: Inherit via back propagation
  Constant10 : Constant  Value=2  OutDataTypeStr=Inherit: Inherit via back propagation
  Constant12 : Constant  Value=3  OutDataTypeStr=Inherit: Inherit via back propagation
  Constant13 : Constant  Value=3  OutDataTypeStr=Inherit: Inherit via back propagation
  Constant{2,6,9,14,17,23,26,30,33,35,37,48} (12 alike) : Constant  Value=WESDem_stCrCtlInhibActv_C
  Constant15 : Constant  Value=2  OutDataTypeStr=Inherit: Inherit via back propagation
  Constant16 : Constant  Value=4  OutDataTypeStr=Inherit: Inherit via back propagation
  Constant{4..5,18..19,31,40..41,49} (8 alike) : Constant  Value=0  OutDataTypeStr=Inherit: Inherit via back propagation
  Constant20 : Constant  Value=WESDem_tiNeutr_C
  Constant21 : Constant  Value=CrCUI_BttnState_conv.CRCUI_SWTOFF  OutDataTypeStr=Inherit: Inherit via back propagation
  Constant22 : Constant  Value=5  OutDataTypeStr=Inherit: Inherit via back propagation
  Constant24 : Constant  Value=CrCUI_BttnState_conv.CRCUI_RES
  Constant25 : Constant  Value=6  OutDataTypeStr=Inherit: Inherit via back propagation
  Constant27 : Constant  Value=3  OutDataTypeStr=Inherit: Inherit via back propagation
  Constant29 : Constant  Value=7  OutDataTypeStr=Inherit: Inherit via back propagation
  Constant3 : Constant  Value=WESDem_tiBlockAftStrt_C
  Constant32 : Constant  Value=8  OutDataTypeStr=Inherit: Inherit via back propagation
  Constant34 : Constant  Value=9  OutDataTypeStr=Inherit: Inherit via back propagation
  Constant36 : Constant  Value=10  OutDataTypeStr=Inherit: Inherit via back propagation
  Constant38 : Constant  Value=WESDem_CalcState_DT
  Constant39 : Constant  Value=WESDem_CalcState_DT
  Constant42 : Constant  Value=8  OutDataTypeStr=Inherit: Inherit via back propagation
  Constant43 : Constant  Value=WESDem_vInhibCrCUI_C  OutMin=0  OutMax=250
  Constant44 : Constant  Value=EISGov_num_conv.ExtDem  OutDataTypeStr=Inherit: Inherit via back propagation
  Constant45 : Constant  Value=11  OutDataTypeStr=Inherit: Inherit via back propagation
  Constant46 : Constant  Value=10  OutDataTypeStr=Inherit: Inherit via back propagation
  Constant47 : Constant  Value=13  OutDataTypeStr=Inherit: Inherit via back propagation
  Constant50 : Constant  Value=7  OutDataTypeStr=Inherit: Inherit via back propagation
  Constant52 : Constant  Value=CrCUI_BttnState_conv.CRCUI_NEUTR
  Constant53 : Constant  Value=CrCUI_BttnState_conv.CRCUI_NEUTR
  Data Type Conversion : DataTypeConversion
  Data Type Conversion1 : DataTypeConversion
  Delay : Delay  DelayLength=1  InitialCondition=0
  Delay1 : Delay  DelayLength=1
  Delay2 : Delay  DelayLength=1  InitialCondition=CrCUI_BttnState_conv.CRCUI_NEUTR
  Delay3 : Delay  DelayLength=1
  Enabled Subsystem : Subsystem  TreatAsAtomicUnit=on
  Enabled Subsystem1 : Subsystem  TreatAsAtomicUnit=on
  GetBit{,1..11,13..16} (16 alike) : CXLib/GetBit  dataTypeString=uint16  dataLength=0
      settings: AttributesFormatString=Get bit from %<dataTypeString>
  Logical Operator{,2,4,7..9,13..14,17..23,28,30..31,37} (19 alike) : Logic  AllPortsSameDT=off  OutDataTypeStr=boolean
  Logical Operator1 : Logic  Operator=NOT  AllPortsSameDT=off  OutDataTypeStr=boolean
  Logical Operator{5,10,15,29} (4 alike) : Logic  Operator=OR  AllPortsSameDT=off  OutDataTypeStr=boolean
  Logical Operator11 : Logic  Operator=NOT  AllPortsSameDT=off  OutDataTypeStr=boolean
  Logical Operator{6,12,16,27} (4 alike) : Logic  Inputs=3  AllPortsSameDT=off  OutDataTypeStr=boolean
  Logical Operator3 : Logic  Operator=NOT  AllPortsSameDT=off  OutDataTypeStr=boolean
  Logical Operator32 : Logic  Operator=OR  Inputs=10  AllPortsSameDT=off  OutDataTypeStr=boolean
  Logical Operator35 : Logic  Operator=OR  Inputs=3  AllPortsSameDT=off  OutDataTypeStr=boolean
  Logical Operator38 : Logic  Operator=OR  Inputs=3  AllPortsSameDT=off  OutDataTypeStr=boolean
  RSFlipFlop : CXLib/RSFlipFlop
  RSFlipFlop1 : CXLib/RSFlipFlop
  RSFlipFlop2 : CXLib/RSFlipFlop
  Relational Operator{,1..2,4,8..11,15..16,20,23} (12 alike) : RelationalOperator  Operator===  OutDataTypeStr=boolean  RndMeth=Simplest
  Relational Operator12 : RelationalOperator  Operator=>  OutDataTypeStr=boolean  RndMeth=Simplest
  Relational Operator13 : RelationalOperator  OutDataTypeStr=boolean  RndMeth=Simplest
  Relational Operator14 : RelationalOperator  Operator=<=  OutDataTypeStr=boolean  RndMeth=Simplest
  Relational Operator{3,18..19,21} (4 alike) : RelationalOperator  Operator=<  OutDataTypeStr=boolean  RndMeth=Simplest
  Relational Operator22 : RelationalOperator  Operator=~=  OutDataTypeStr=boolean  RndMeth=Simplest
  Relational Operator5 : RelationalOperator  Operator=~=  OutDataTypeStr=boolean  RndMeth=Simplest
  Relational Operator6 : RelationalOperator  Operator=~=  OutDataTypeStr=boolean  RndMeth=Simplest
  Relational Operator7 : RelationalOperator  Operator=~=  OutDataTypeStr=boolean  RndMeth=Simplest  InputSameDT=on
  Scope : Scope
  Switch{,1,3..16} (16 alike) : Switch  Criteria=u2 ~= 0
  Switch2 : Switch  Criteria=u2 ~= 0  InputSameDT=on
  Terminator{,1..3} (4 alike) : Terminator
  TurnOnDelay : CXLib/TurnOnDelay
  TurnOnDelay1 : CXLib/TurnOnDelay
  WESDem_stCrCtl : Outport  Description=State control of the working engine speed demand  OutMin=0  OutMax=65535  OutDataTypeStr=State_uint16
  wires:
  Constant/1 -> RSFlipFlop/1
  Constant3/1 -> TurnOnDelay/2
  TurnOnDelay/1 -> RSFlipFlop/2
  RSFlipFlop/1 -> Logical Operator/1
  RSFlipFlop/2 -> Terminator/1
  Constant2/1 -> GetBit/1
  GetBit/1 -> Logical Operator/2
  Constant4/1 -> GetBit/2
  Logical Operator/1 -> Switch4/2, Logical Operator38/2, Logical Operator35/1
  WESDem_stShutOff/1 -> Delay/1, Relational Operator/1
  Constant5/1 -> Relational Operator/2
  Relational Operator/1 -> Logical Operator9/1, Logical Operator6/1, Logical Operator1/1
  Logical Operator1/1 -> Logical Operator2/1
  Constant6/1 -> GetBit1/1
  GetBit1/1 -> Logical Operator2/2
  Constant7/1 -> GetBit1/2
  Logical Operator2/1 -> Switch3/2, Logical Operator38/1, Logical Operator35/2
  WESDem_stCfg/1 -> [WESDem_stCfg], GetBit2/1
  Constant8/1 -> GetBit2/2
  GetBit2/1 -> Logical Operator3/1
  Constant9/1 -> GetBit3/1
  GetBit3/1 -> Logical Operator4/2
  Constant10/1 -> GetBit3/2
  Logical Operator3/1 -> Logical Operator4/1
  Logical Operator4/1 -> Switch5/2, Logical Operator32/1
  WESDem_stModeChange/1 -> Relational Operator6/1, Relational Operator4/1, Relational Operator2/1, Relational Operator1/1
  Constant11/1 -> Relational Operator1/2
  Constant12/1 -> Relational Operator2/2
  Relational Operator1/1 -> Logical Operator5/1
  Relational Operator2/1 -> Logical Operator5/2
  Logical Operator5/1 -> Logical Operator6/2
  VehV_v/1 -> [VehV], Relational Operator3/1
  WESDem_vMaxActv/1 -> [WESDem_vMaxActv], Relational Operator3/2
  Relational Operator3/1 -> Logical Operator6/3
  Constant14/1 -> GetBit4/1
  GetBit4/1 -> Logical Operator8/2
  Constant13/1 -> GetBit4/2
  Logical Operator6/1 -> Logical Operator8/1
  Logical Operator8/1 -> Switch6/2, Switch1/2
  Constant15/1 -> Relational Operator4/2
  Constant17/1 -> GetBit5/1
  GetBit5/1 -> Logical Operator7/2
  Constant16/1 -> GetBit5/2
  Relational Operator4/1 -> Logical Operator7/1
  Logical Operator7/1 -> Switch7/2, Logical Operator38/3, Logical Operator35/3
  Constant18/1 -> Relational Operator5/2
  Delay/1 -> Relational Operator5/1
  Relational Operator5/1 -> Logical Operator9/2
  Constant19/1 -> Relational Operator6/2
  Relational Operator6/1 -> Logical Operator10/2
  Logical Operator9/1 -> Logical Operator10/1
  Logical Operator10/1 -> Logical Operator11/1, RSFlipFlop1/1
  Logical Operator11/1 -> TurnOnDelay1/1
  Constant20/1 -> TurnOnDelay1/2
  TurnOnDelay1/1 -> RSFlipFlop1/2
  RSFlipFlop1/1 -> Logical Operator12/1
  Constant21/1 -> Relational Operator7/2
  Relational Operator7/1 -> Logical Operator12/2
  Constant23/1 -> GetBit6/1
  GetBit6/1 -> Logical Operator12/3
  Constant22/1 -> GetBit6/2
  Logical Operator12/1 -> Switch8/2, Logical Operator32/2
  Constant24/1 -> Relational Operator8/2
  Relational Operator8/1 -> Logical Operator20/1, Logical Operator18/1, Logical Operator16/1, Logical Operator13/1
  Relational Operator16/1 -> Logical Operator13/2
  Constant26/1 -> GetBit7/1
  GetBit7/1 -> Logical Operator14/2
  Constant25/1 -> GetBit7/2
  Logical Operator13/1 -> Logical Operator14/1
  Logical Operator14/1 -> Switch9/2, Logical Operator32/3
  Brk_st/1 -> Relational Operator10/1, Relational Operator9/1
  Constant27/1 -> Relational Operator9/2
  Constant28/1 -> Relational Operator10/2
  Relational Operator9/1 -> Logical Operator15/1
  Relational Operator10/1 -> Logical Operator15/2
  Logical Operator15/1 -> Logical Operator16/2
  Constant30/1 -> GetBit8/1
  GetBit8/1 -> Logical Operator17/2
  Constant29/1 -> GetBit8/2
  Logical Operator17/1 -> Switch10/2, Logical Operator32/4
  Logical Operator16/1 -> Logical Operator17/1
  "WESDem_stMode "/1 -> Relational Operator11/1
  Constant31/1 -> Relational Operator11/2
  Relational Operator11/1 -> Logical Operator16/3
  Relational Operator15/1 -> Logical Operator18/2
  Constant33/1 -> GetBit9/1
  GetBit9/1 -> Logical Operator19/2
  Constant32/1 -> GetBit9/2
  Logical Operator19/1 -> Switch11/2, Logical Operator32/5
  Logical Operator18/1 -> Logical Operator19/1
  CoEng_stEngStop/1 -> Logical Operator20/2
  Constant35/1 -> GetBit10/1
  GetBit10/1 -> Logical Operator21/2
  Constant34/1 -> GetBit10/2
  Logical Operator21/1 -> Switch12/2, Logical Operator32/6
  Logical Operator20/1 -> Logical Operator21/1
  "WESDem_vMaxAcc_mp "/1 -> Relational Operator14/2, Relational Operator12/2
  Constant37/1 -> GetBit11/1
  GetBit11/1 -> Logical Operator22/2
  Constant36/1 -> GetBit11/2
  Logical Operator22/1 -> Switch13/2, Logical Operator32/7
  Relational Operator12/1 -> Logical Operator22/1
  [WESDem_vMaxActv] -> Relational Operator18/2, Relational Operator13/2
  Relational Operator13/1 -> Logical Operator23/1
  Relational Operator14/1 -> Logical Operator23/2
  Enabled Subsystem/1("WESDem_stCrCtlInhib_mp.11 ") -> Switch14/2, Logical Operator32/8
  Enabled Subsystem1/1("WESDem_stCrCtlInhib_mp.12 ") -> Switch15/2, Logical Operator32/9
  Constant42/1 -> GetBit13/2
  Constant43/1 -> Relational Operator19/2
  "EISGov_numCurrFunc "/1 -> Relational Operator20/1
  Constant44/1 -> Relational Operator20/2
  GetBit13/1 -> Logical Operator27/1
  Relational Operator19/1 -> Logical Operator27/2
  Constant45/1 -> GetBit14/2
  CoETS_stTSEATrqSpdReq/1 -> GetBit15/1, GetBit14/1
  Constant46/1 -> GetBit15/2
  EISGov_trq/1 -> Relational Operator21/1
  GlbDa_trqSpdGovRed/1 -> Relational Operator21/2
  GetBit15/1 -> Logical Operator28/1
  Relational Operator21/1 -> Logical Operator28/2
  GetBit14/1 -> Logical Operator29/1
  Logical Operator28/1 -> Logical Operator29/2
  Relational Operator20/1 -> Logical Operator30/1
  Logical Operator29/1 -> Logical Operator30/2
  Logical Operator30/1 -> Logical Operator27/3
  Constant48/1 -> GetBit16/1
  GetBit16/1 -> Logical Operator31/2
  Constant47/1 -> GetBit16/2
  Logical Operator31/1 -> Switch16/2, Logical Operator32/10
  Logical Operator27/1 -> Logical Operator31/1
  Data Type Conversion/1 -> Switch/3  "WESDem_stCrCtlRaw_mp"
  Logical Operator32/1 -> Switch/2
  Switch1/1 -> Switch2/3
  Logical Operator35/1 -> Scope/1, Switch2/2
  Switch2/1 -> WESDem_stCrCtl/1
  CrCUI_stBttn/1 -> Relational Operator8/1, Delay2/1, Relational Operator22/1, Data Type Conversion/1, Relational Operator7/1, Enabled Subsystem/1(CrCUI_stBttn)
  Constant52/1 -> Relational Operator22/2
  Constant53/1 -> Relational Operator23/2
  Relational Operator22/1 -> Logical Operator37/1
  Relational Operator23/1 -> Logical Operator37/2
  Logical Operator37/1 -> RSFlipFlop2/1
  Logical Operator38/1 -> RSFlipFlop2/2
  RSFlipFlop2/2 -> Terminator1/1
  Delay2/1 -> Relational Operator23/1
  "WESDem_stCrCtl "/1 -> Enabled Subsystem/3("WESDem_stCrCtl ")
  [WESDem_stCrCtlNeutrChng_mp] -> Enabled Subsystem1/2("WESDem_stCrCtlNeutrChng_mp ")
  RSFlipFlop1/2 -> Terminator3/1
  Constant38/1 -> TurnOnDelay/3
  Constant39/1 -> TurnOnDelay1/3
  RSFlipFlop2/1 -> [WESDem_stCrCtlNeutrChng_mp]  "WESDem_stCrCtlNeutrChng_mp"
  Bit Clear/1 -> Switch4/3
  Bit Set/1 -> Switch4/1
  Switch4/1 -> Bit Clear1/1, Bit Set1/1
  Bit Clear1/1 -> Switch3/3
  Bit Set1/1 -> Switch3/1
  Switch3/1 -> Bit Clear2/1, Bit Set2/1
  Bit Clear2/1 -> Switch5/3
  Bit Set2/1 -> Switch5/1
  Switch/1 -> Switch1/3
  Constant50/1 -> Switch1/1
  Constant49/1 -> Switch/1
  Constant51/1 -> Switch2/1
  Bit Clear3/1 -> Switch6/3
  Bit Set3/1 -> Switch6/1
  Switch5/1 -> Bit Clear3/1, Bit Set3/1
  Bit Clear4/1 -> Switch7/3
  Bit Set4/1 -> Switch7/1
  Switch6/1 -> Bit Clear4/1, Bit Set4/1
  Bit Clear5/1 -> Switch8/3
  Bit Set5/1 -> Switch8/1
  Switch7/1 -> Bit Clear5/1, Bit Set5/1
  Bit Clear6/1 -> Switch9/3
  Bit Set6/1 -> Switch9/1
  Switch8/1 -> Bit Clear6/1, Bit Set6/1
  Bit Clear7/1 -> Switch10/3
  Bit Set7/1 -> Switch10/1
  Switch9/1 -> Bit Clear7/1, Bit Set7/1
  Bit Clear8/1 -> Switch11/3
  Bit Set8/1 -> Switch11/1
  Switch10/1 -> Bit Clear8/1, Bit Set8/1
  Bit Clear9/1 -> Switch12/3
  Bit Set9/1 -> Switch12/1
  Switch11/1 -> Bit Clear9/1, Bit Set9/1
  Bit Clear10/1 -> Switch13/3
  Bit Set10/1 -> Switch13/1
  Switch12/1 -> Bit Clear10/1, Bit Set10/1
  Bit Clear11/1 -> Switch14/3
  Bit Set11/1 -> Switch14/1
  Switch13/1 -> Bit Clear11/1, Bit Set11/1
  Bit Clear12/1 -> Switch15/3
  Bit Clear13/1 -> Switch16/3
  Bit Set13/1 -> Switch16/1
  Switch16/1 -> Delay3/1, Terminator2/1  "WESDem_stCrCtlInhib_mp"
  Switch15/1 -> Bit Clear13/1, Bit Set13/1
  Constant1/1 -> Delay1/1
  Data Type Conversion1/1 -> TurnOnDelay/1
  Delay1/1 -> Data Type Conversion1/1
  Delay3/1 -> Bit Clear/1, Bit Set/1
  [WESDem_stCfg] -> GetBit13/1
  [VehV] -> Relational Operator19/1, Relational Operator18/1, Relational Operator14/1, Relational Operator13/1, Relational Operator12/1
  Logical Operator23/1 -> Enabled Subsystem/2(enable)
  Relational Operator18/1 -> Enabled Subsystem1/1("enable ")
  Bit Set12/1 -> Switch15/1
  Switch14/1 -> Bit Clear12/1, Bit Set12/1
  "DSM_bstFId_WESDemBrkClth "/1 -> Relational Operator15/2
  Constant40/1 -> Relational Operator15/1
  "DSM_btFId_WESDemVehSpdSens "/1 -> Relational Operator16/2
  Constant41/1 -> Relational Operator16/1

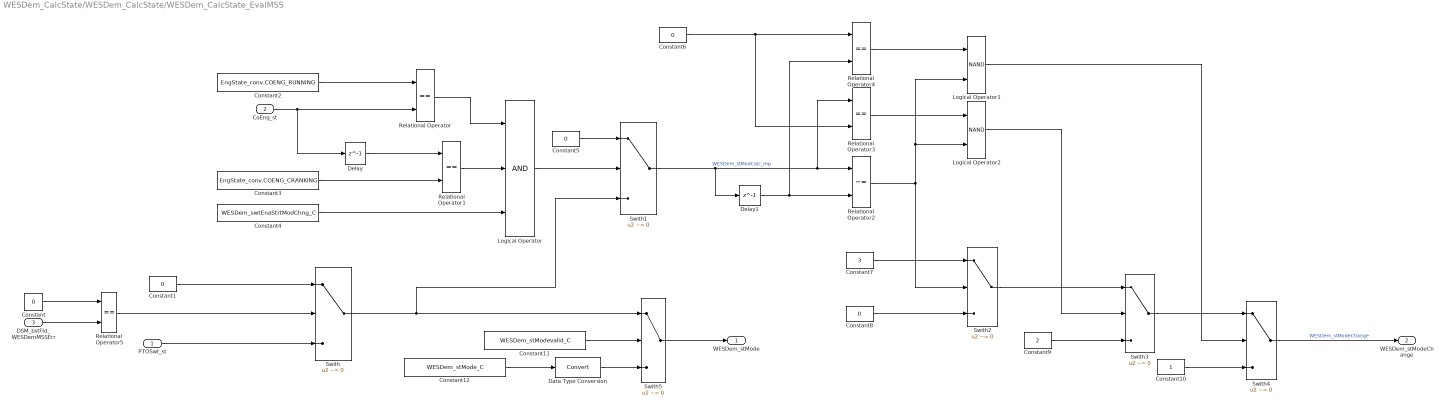
== system WESDem_CalcState/WESDem_CalcState/WESDem_CalcState_EvalMSS ==
  PTOSwt_st : Inport  Description=Power Take-off switch's current state for a specific input voltage  OutMin=0  OutMax=255  OutDataTypeStr=State_uint8
  CoEng_st : Inport  Description=Engine coordinator state  Port=2  OutDataTypeStr=Enum: EngState_conv
  "DSM_bstFId_WESDemMSSErr " : Inport  Description=Function Identifier for WESDem reactions in case of multiple state switch error  Port=3  OutMin=0  OutMax=1  OutDataTypeStr=boolean
  Constant{,1,5..6} (4 alike) : Constant  Value=0  OutDataTypeStr=Inherit: Inherit via back propagation
  Constant10 : Constant  OutDataTypeStr=State_uint8
  Constant11 : Constant  Value=WESDem_stModevalid_C
  Constant12 : Constant  Value=WESDem_stMode_C
  Constant2 : Constant  Value=EngState_conv.COENG_RUNNING
  Constant3 : Constant  Value=EngState_conv.COENG_CRANKING
  Constant4 : Constant  Value=WESDem_swtEnaStrtModChng_C
  Constant7 : Constant  Value=3  OutDataTypeStr=State_uint8
  Constant8 : Constant  Value=0  OutDataTypeStr=State_uint8
  Constant9 : Constant  Value=2  OutDataTypeStr=State_uint8
  Data Type Conversion : DataTypeConversion
  Delay : Delay  DelayLength=1  InitialCondition=EngState_conv.COENG_STANDBY
  Delay1 : Delay  DelayLength=1  InitialCondition=0
  Logical Operator : Logic  Inputs=3  AllPortsSameDT=off  OutDataTypeStr=boolean
  Logical Operator1 : Logic  Operator=NAND  AllPortsSameDT=off  OutDataTypeStr=boolean
  Logical Operator2 : Logic  Operator=NAND  AllPortsSameDT=off  OutDataTypeStr=boolean
  Relational Operator{,1,3..5} (5 alike) : RelationalOperator  Operator===  OutDataTypeStr=boolean  RndMeth=Simplest
  Relational Operator2 : RelationalOperator  Operator=~=  OutDataTypeStr=boolean  RndMeth=Simplest
  Swith{,1..5} (6 alike) : Switch  Criteria=u2 ~= 0
  WESDem_stMode : Outport  Description=Operating mode of the working engine speed demand  OutMin=0  OutMax=255  OutDataTypeStr=State_uint8
  WESDem_stModeChange : Outport  Description=Operating mode change of the working engine speed demand  Port=2  OutMin=0  OutMax=255  OutDataTypeStr=State_uint8
  wires:
  Constant3/1 -> Relational Operator1/2
  Constant9/1 -> Swith3/3
  Relational Operator3/1 -> Logical Operator2/1
  Relational Operator2/1 -> Logical Operator1/2, Logical Operator2/2, Swith2/2
  Relational Operator4/1 -> Logical Operator1/1
  Swith2/1 -> Swith3/1
  Constant8/1 -> Swith2/3
  Logical Operator1/1 -> Swith4/2
  Constant4/1 -> Logical Operator/3
  Swith1/1 -> Delay1/1, Relational Operator3/1, Relational Operator2/1  "WESDem_stModCalc_mp"
  Relational Operator1/1 -> Logical Operator/2
  Constant5/1 -> Swith1/1
  Swith/1 -> Swith1/3, Swith5/1
  Swith4/1 -> WESDem_stModeChange/1  "WESDem_stModeChange"
  Relational Operator5/1 -> Swith/2
  Constant6/1 -> Relational Operator3/2, Relational Operator4/1
  Swith3/1 -> Swith4/1
  Logical Operator2/1 -> Swith3/2
  Delay1/1 -> Relational Operator4/2, Relational Operator2/2
  Logical Operator/1 -> Swith1/2
  Constant7/1 -> Swith2/1
  Constant10/1 -> Swith4/3
  PTOSwt_st/1 -> Swith/3
  Relational Operator/1 -> Logical Operator/1
  Constant2/1 -> Relational Operator/1
  Constant1/1 -> Swith/1
  CoEng_st/1 -> Delay/1, Relational Operator/2
  Delay/1 -> Relational Operator1/1
  Swith5/1 -> WESDem_stMode/1
  Constant11/1 -> Swith5/2
  Constant12/1 -> Data Type Conversion/1
  Data Type Conversion/1 -> Swith5/3
  "DSM_bstFId_WESDemMSSErr "/1 -> Relational Operator5/2
  Constant/1 -> Relational Operator5/1
